simulink model "hydraulic_tank_system"  (R2021a)
settings: Solver=VariableStepAuto  StartTime=0.0  StopTime=600  RelTol=1e-3
values from neighbouring files (symbols this model uses):
  A1 = 0.01    [run_hydraulic_tank_system.m]
  a1 = 0.2*(10^-4)    (= 2e-05)    [run_hydraulic_tank_system.m]
  A2 = A1    (= 0.01)    [run_hydraulic_tank_system.m]
  a2 = 0.32*(10^-4)    (= 3.2e-05)    [run_hydraulic_tank_system.m]
  amp = 3    [run_hydraulic_tank_system.m]
  C1 = 12    [run_hydraulic_tank_system.m]
  C2 = C1    (= 12)    [run_hydraulic_tank_system.m]
  kp = 15*(10^-6)    (= 1.5e-05)    [run_hydraulic_tank_system.m]
settings Model: Creator=cop20skj  LastModifiedBy=cop20skj

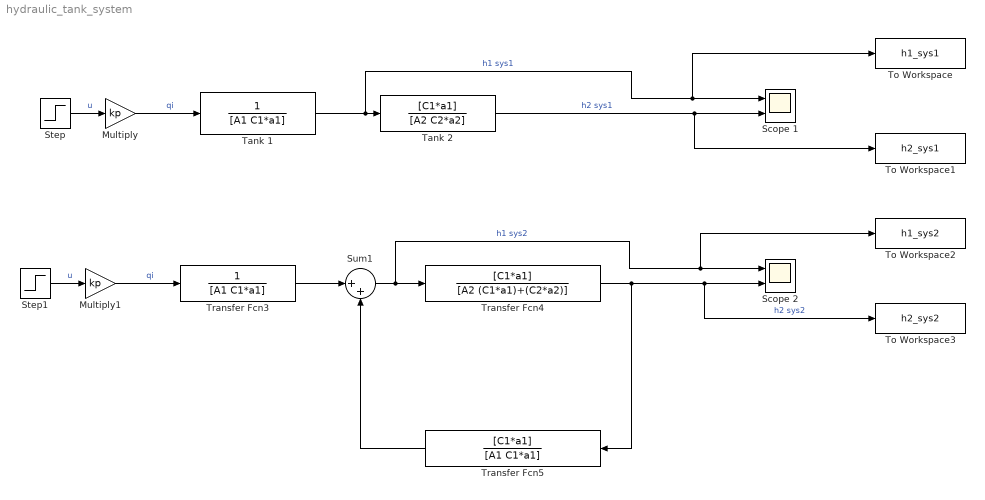
== system hydraulic_tank_system ==
  Multiply : Gain  Gain=kp
  Multiply1 : Gain  Gain=kp
  Scope 1 : Scope  NumInputPorts=2
  Scope 2 : Scope  NumInputPorts=2
  Step : Step  After=amp  SampleTime=0
  Step1 : Step  After=amp  SampleTime=0
  Sum1 : Sum  Inputs=|++
  Tank 1 : TransferFcn  Denominator=[A1 C1*a1]
  Tank 2 : TransferFcn  Numerator=[C1*a1]  Denominator=[A2 C2*a2]
  To Workspace : ToWorkspace  VariableName=h1_sys1  SaveFormat=Timeseries  SampleTime=-1
  To Workspace1 : ToWorkspace  VariableName=h2_sys1  SaveFormat=Timeseries  SampleTime=-1
  To Workspace2 : ToWorkspace  VariableName=h1_sys2  SaveFormat=Timeseries  SampleTime=-1
  To Workspace3 : ToWorkspace  VariableName=h2_sys2  SaveFormat=Timeseries  SampleTime=-1
  Transfer Fcn3 : TransferFcn  Denominator=[A1 C1*a1]
  Transfer Fcn4 : TransferFcn  Numerator=[C1*a1]  Denominator=[A2 (C1*a1)+(C2*a2)]
  Transfer Fcn5 : TransferFcn  Numerator=[C1*a1]  Denominator=[A1 C1*a1]
  wires:
  Multiply/1 -> Tank 1/1  "qi"
  Multiply1/1 -> Transfer Fcn3/1  "qi"
  Step/1 -> Multiply/1  "u"
  Tank 1/1 -> Scope 1/1, To Workspace/1, Tank 2/1  "h1 sys1"
  Step1/1 -> Multiply1/1  "u"
  Transfer Fcn3/1 -> Sum1/1
  Sum1/1 -> Scope 2/1, To Workspace2/1, Transfer Fcn4/1  "h1 sys2"
  Transfer Fcn5/1 -> Sum1/2
  Transfer Fcn4/1 -> Scope 2/2, To Workspace3/1, Transfer Fcn5/1  "h2 sys2"
  Tank 2/1 -> Scope 1/2, To Workspace1/1  "h2 sys1"
